simulink model "Traffic_Light"  (R2016a)
settings: Solver=FixedStepDiscrete  StartTime=0.0  StopTime=inf  RelTol=1e-3
settings Model: Creator=Muhammed  LastModifiedBy=Muhammed
settings OptimizationCC: DefaultParameterBehavior=Inlined  InlineInvariantSignals=on  EnableMemcpy=off  OptimizeModelRefInitCode=on  LifeSpan=1
settings DebuggingCC: UnderspecifiedInitializationDetection=Classic  MergeDetectMultiDrivingBlocksExec=none
settings ModelReferenceCC: PropagateSignalLabelsOutOfModel=off
settings RTWCC: SystemTargetFile=ert.tlc  GenCodeOnly=on  TemplateMakefile=ert_default_tmf  GenerateReport=on  IncludeHyperlinkInReport=on  LaunchReport=on  GenerateTraceInfo=on  GenerateTraceReport=on  GenerateTraceReportSl=on  GenerateTraceReportSf=on  GenerateTraceReportEml=on
settings CodeAppCC: ForceParamTrailComments=on  IgnoreCustomStorageClasses=off  OperatorAnnotations=on  SimulinkDataObjDesc=on  SFDataObjDesc=on  MATLABFcnDesc=on  InsertBlockDesc=on  MATLABSourceComments=on
settings ERTTargetCC: GenerateSampleERTMain=on  InlinedParameterPlacement=NonHierarchical  ERTCustomFileTemplate=example_file_process.tlc

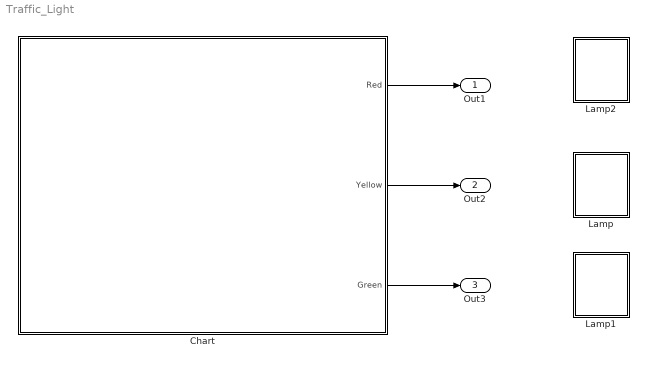
== system Traffic_Light ==
  Chart : Stateflow chart  TreatAsAtomicUnit=on
  Lamp : Subsystem  DialogController=hmiCreateDDGDialog  IsWebBlock=on  mask(MWDashboardBlock){webBlockId=3bf1d0c1-2f43-47bd-8468-30b07416ff45, webBlockType=lamp, ShowInLibBrowser=on, ShowInitialText=on, HMISrcModelName=Traffic_Light}
      mask prompts: webBlockType "WebBlock Type"; HMISrcModelName "Source Model"
      mask Help: helpview([docroot '/mapfiles/simulink.map'], 'hmi_lamp')
      mask Display:
      | if strcmp(get_param(bdroot(gcb),'BlockDiagramType'), 'library')
      |     image([(matlabroot) '/toolbox/simulink/hmi/icons/Lamp.png']);
      | end
  Lamp1 : Subsystem  DialogController=hmiCreateDDGDialog  IsWebBlock=on  mask(MWDashboardBlock){webBlockId=5bd0aad9-9833-42f6-83ac-ea4802cf318a, webBlockType=lamp, ShowInLibBrowser=on, ShowInitialText=on, HMISrcModelName=Traffic_Light}
      mask prompts: webBlockType "WebBlock Type"; HMISrcModelName "Source Model"
      mask Help: helpview([docroot '/mapfiles/simulink.map'], 'hmi_lamp')
      mask Display:
      | if strcmp(get_param(bdroot(gcb),'BlockDiagramType'), 'library')
      |     image([(matlabroot) '/toolbox/simulink/hmi/icons/Lamp.png']);
      | end
  Lamp2 : Subsystem  DialogController=hmiCreateDDGDialog  IsWebBlock=on  mask(MWDashboardBlock){webBlockId=7e686a7b-aed4-42fa-80d7-cdf83f188e34, webBlockType=lamp, ShowInLibBrowser=on, ShowInitialText=on, HMISrcModelName=Traffic_Light}
      mask prompts: webBlockType "WebBlock Type"; HMISrcModelName "Source Model"
      mask Help: helpview([docroot '/mapfiles/simulink.map'], 'hmi_lamp')
      mask Display:
      | if strcmp(get_param(bdroot(gcb),'BlockDiagramType'), 'library')
      |     image([(matlabroot) '/toolbox/simulink/hmi/icons/Lamp.png']);
      | end
  Out1 : Outport
  Out2 : Outport  Port=2
  Out3 : Outport  Port=3
  wires:
  Chart/1(Red) -> Out1/1
  Chart/3(Green) -> Out3/1
  Chart/2(Yellow) -> Out2/1

== system Traffic_Light/Lamp ==

== system Traffic_Light/Lamp1 ==

== system Traffic_Light/Lamp2 ==

== stateflow chart Traffic_Light/Chart ==
  state Go
    en:
    Red=0;
    Yellow=0;
    Green=0;
    du:
    Red=0;
    Yellow=0;
    Green=1;
    ex:
  state Stop
    en:
    Red=0;
    Yellow=0;
    Green=0;
    du:
    Red=1;
    Yellow=0;
    Green=0;
    ex:
  state Ready
    en:
    Red=0;
    Yellow=0;
    Green=0;
    du:
    Red=0;
    Yellow=1;
    Green=0;
    ex:
  (default) -> Stop
  Go -> Stop : after(3000,msec)
  Stop -> Ready : after(3000,msec)
  Ready -> Go : after(3000,msec)
  data: Red output uint8; Yellow output uint8; Green output uint8
